simulink model "ds_fivezoneg36_backup"  (R2020a)
settings: Solver=ode1be  StartTime=182*24*3600  StopTime=183*24*3600  FixedStep=0.001  RelTol=1e-3
PostLoadFcn:
  | if any(exist('dsrtsu_mdlpostloadfcn', 'file') ~= 0), dsrtsu_mdlpostloadfcn('Execute', bdroot); end
InitFcn:
  | , if any(exist('rtifpga_mdlclblib', 'file') ~= 0), rtifpga_mdlclblib('Init', bdroot); end,
undefined symbols (not defined in the file or in its folder): dspaceexample_f_dy975f7hquM
libraries: neural x7
settings Model: DSRTSU_INTERNAL_RTI_VER=560  DSRTSU_INTERNAL_RTI_TYPE=rti1401  RTICANMMDATA=struct('GeneralSetupData',struct('modelroot','D:\github\dspace-modelica-example\dSpaceExample','generalsettings',struct('filesettings',struct('destfolder',struct('Name','RTICANMM_FILES','Check',1),'buildfolder',struct('Name','.','Check',1),'AbsDestfolder',struct('Name','D:\github\dspace-modelica-example\dSpaceExample\RTICANMM_FILES'),'AbsBuildfolder',struct('Name','D:\github\dspace-modelica-example\dSpaceExample'))),'options',struct('addpaths',1,'rmpaths',1,'addtrcexclusion',true,'cannavigator',struct('checkmonitoring',0),'show_usrtrc',0,'use_usrtrc',0),'advanced',struct('options',ones(1,100)),'MPSetup',{{}},'RTI',struct('Type','GRT','Ver','','Date',''),'modelname','ds_fivezoneg36','block','ds_fivezoneg36'))  DSRTSU_INTERNAL_RTIFPGA=160  Creator=yangyang.fu  LastModifiedBy=yangyang.fu
settings HardwareCC: TargetIntDivRoundTo=Zero  TargetEndianess=BigEndian  TargetHWDeviceType=Custom Processor->Custom
settings SFSimCC: MATLABDynamicMemAlloc=off
settings RTWCC: Description=Generic Real-Time Target  CustomInclude="\"C:\\Program Files\\Dymola 2021\\Source\""
settings GRTTargetCC: TargetLangStandard=C89/C90 (ANSI)

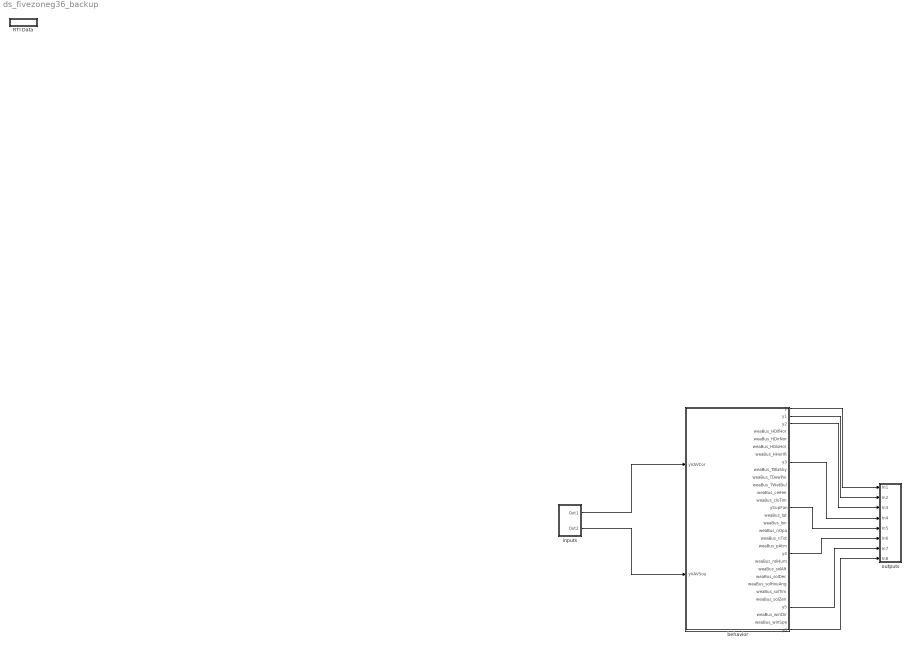
== system ds_fivezoneg36_backup ==
  RTI Data : Subsystem  Tag=struct('RTIDataServer',struct('RTIDataServerVs','2','RTIModelDescription','struct(''main'',''ds_fivezoneg36'',''sub'','''',''isMp'',0)'))  LoadFcn="if exist('rtidc'), try,  rtidc('DataHostBlockClbLoad', gcbh); catch, disp(['Warning: ''LoadFcn'' for RTI Data block failed: ' lasterr]); end, end,"  mask(RTI_DATA_HOST){}
      mask help:
      | RTI Data Block.
      | This block is used by RTI to store internal model-dependent data.
      | Please keep this block on the root level of the model. Deleting this block will result in data loss.
      |
      | NEVER DELETE OR COPY THIS BLOCK!
      settings: CopyFcn="if exist('rtidc'), try,  rtidc('DataHostBlockClbCopy', gcbh); catch, disp(['Warning: ''CopyFcn'' for RTI Data block failed: ' lasterr]); end, end,"  DeleteFcn="if exist('rtidc'), try,  rtidc('DataHostBlockClbDelete', gcbh); catch, disp(['Warning: ''DeleteFcn'' for RTI Data block failed: ' lasterr]); end, end,"  ModelCloseFcn="if exist('rtidc'), try,  rtidc('DataHostBlockClbModelClose', gcbh); catch, disp(['Warning: ''ModelCloseFcn'' for RTI Data block failed: ' lasterr]); end, end,"  PreSaveFcn="if exist('rtidc'), try,  rtidc('DataHostBlockClbPreSave', gcbh); catch, disp(['Warning: ''PreSaveFcn'' for RTI Data block failed: ' lasterr]); end, end,"  PostSaveFcn="if exist('rtidc'), try,  rtidc('DataHostBlockClbPostSave', gcbh); catch, disp(['Warning: ''PostSaveFcn'' for RTI Data block failed: ' lasterr]); end, end,"  NameChangeFcn="if exist('rtidc'), try,  rtidc('DataHostBlockClbNameChange', gcbh); catch, disp(['Warning: ''NameChangeFcn'' for RTI Data block failed: ' lasterr]); end, end,"
      mask Help:
      | RTI Data Block.
      | This block is used by RTI to store internal model-dependent data.
      | Please keep this block on the root level of the model. Deleting this block will result in data loss.
      | 
      | NEVER DELETE OR COPY THIS BLOCK!
      mask Display:
      | text(0.5, 0.5, 'RTI Data', 'HorizontalAlignment', 'center');
      | plot([1 0]);
  behavior : Subsystem
  inputs : Subsystem
  outputs : Subsystem
  wires:
  inputs/1(Out1) -> behavior/1(yVAVCor)
  inputs/2(Out2) -> behavior/2(yVAVSou)
  behavior/1(y) -> outputs/1(In1)
  behavior/2(y1) -> outputs/2(In2)
  behavior/3(y2) -> outputs/3(In3)
  behavior/8(y3) -> outputs/4(In4)
  behavior/14(ySupFan) -> outputs/5(In5)
  behavior/20(y4) -> outputs/6(In6)
  behavior/27(y5) -> outputs/7(In7)
  behavior/30(y6) -> outputs/8(In8)

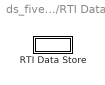
== system ds_fivezoneg36_backup/RTI Data ==
  RTI Data Store : Subsystem  Tag=struct('private',struct('version',struct('dsVer',uint32(2),'dsVerCreation',uint32(2),'RTI',struct('ver','7.14','type','RTI1401')),'access',struct('type','Model','isPerm',1,'created',['22-Sep-2021 20:42:39'],'modified',['29-Sep-2021 14:30:35'],'location','')),'public',struct('main',struct('data',[]),'sub',struct('name','','data',[])))  mask(RTI_DATA_STORE){}
      mask help:
      | RTI Data Store Block. This block is used by RTI to store internal model dependent data. Deleting this block will result in data loss.
      |
      | NEVER DELETE, COPY, OR MODIFY THIS BLOCK!
      mask Help:
      | RTI Data Store Block. This block is used by RTI to store internal model dependent data. Deleting this block will result in data loss.
      | 
      | NEVER DELETE, COPY, OR MODIFY THIS BLOCK!
      mask Display: text(0.5, 0.5, ' ', 'HorizontalAlignment', 'center');

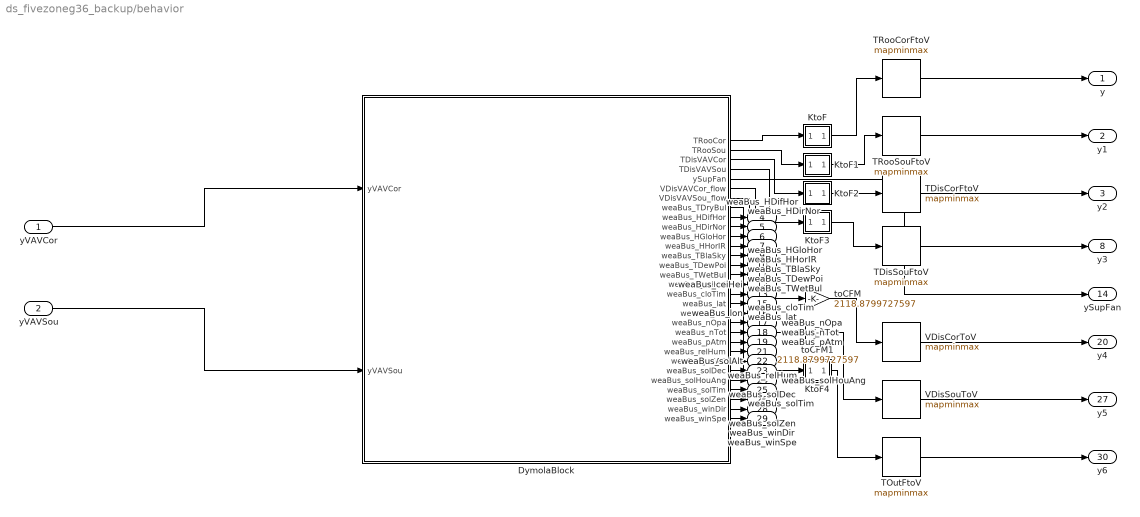
== system ds_fivezoneg36_backup/behavior ==
  yVAVCor : Inport
  yVAVSou : Inport  Port=2
  DymolaBlock : Subsystem  Tag=07-Sep-2021 15:30:30#975  LoadFcn=if exist('newDymolaGui') newDymolaGui('ds_fivezoneg36/behavior/DymolaBlock','PostLoadNew'); else error('Dymola not installed. Must install at least the file newDymolaGui.p'); end;
      mask help:
      | Dymola block.
      | A dymola block allows acausal physical modeling.
      | See Dymola manual for usage.
      settings: CopyFcn=newDymolaGui('07-Sep-2021 15:30:30#975','Copy');  DeleteFcn=if exist('newDymolaGui') newDymolaGui('ds_fivezoneg36/behavior/DymolaBlock','Delete'); end;  NameChangeFcn=newDymolaGui('07-Sep-2021 15:30:30#975','Copy');  OpenFcn=newDymolaGui('ds_fivezoneg36/behavior/DymolaBlock','Init');
      mask Display: image(reshape([1;1;1;1;1;1;1;1;1;1;1;1;1;1;1;1;1;1;1;1;1;1;0;0;0;0;0;0;0;0;0;0;1;1;1;1;1;1;1;1;0;1;1;1;1;1;1;1;1;0;1;1;1;1;1;0;0;0;0;0;0;0;1;1;0;0;0;0;0;0;0;1;1;0;0;0;0;0;0;0;1;1;0;0;0;0;0;0;0;1;1;0;0;0;0;0;0;0;1;1;0;0;0;0;0;0;0;1;1;0;0;0;0;0;0;0;1;1;0;0;0;0;0;0;0;1;1;0;0;0;0;0;0;0;1;1;0;0;0;0;0;0;0;1;1;0;0;0;0;0;0;0;1;1;0;0;0;0;0;0;0;1;1;0;0;0;0;0;0;0;1;1;0;0;0;0;0;0;0;1;1;0;0;0;0;0;0;0;1;1;0;0;0;0;0;0;0;1;1;0;0;0;0;0;0;0;1;1;0;0;0;0;0;0;0;1;1;0;0;0;0;0;0;0;1;1;0;0;0;0;0;0;0;1;1;0;0;0;0;0;0;0;1;1;0;0;0;0;0;0;0;1;1;0;0;0;0;0;0;0;1;1;0;0;0;0;0;0;0;1;1;1;1;1;0;1;1;1;1;1;1;1;1;0;1;1;1;1;1;1;1;1;0;0;0;0;0;0;0;0;0;0;1;1;1;1;1;1;1;1;1;1;1;1;1;1;1;1;1;1;1;1;1;1;1;1;1;1;1;1;1;1;1;1;1;1;1;1;1;1;1;1;1;1;1;1;0;0;0;0;0;0;0;0;0;0;1;1;1;1;1;1;1;1;0;1;1;1;1;1;1;1;1;0;1;1;1;1;1;0;0;0;0;0;0;0;1;1;0;0;0;0;0;0;0;1;1;0;0;0;0;0;0;0;1;1;0;0;0;0;0;0;0;1;1;0;0;0;0;0;0;0;1;1;0;0;0;0;0;0;0;1;1;0;0;0;0;0;0;0;1;1;0;0;0;0;0;0;0;1;1;0;0;0;0;0;0;0;1;1;0;0;0;0;0;0;0;1;1;0;0;0;0;0;0;0;1;1;0;0;0;0;0;0;0;1;1;0;0;0;0;0;0;0;1;1;0;0;0;0;0;0;0;1;1;0;0;0;0;0;0;0;1;1;0;0;0;0;0;0;0;1;1;0;0;0;0;0;0;0;1;1;0;0;0;0;0;0;0;1;1;0;0;0;0;0;0;0;1;1;0;0;0;0;0;0;0;1;1;0;0;0;0;0;0;0;1;1;0;0;0;0;0;0;0;1;1;0;0;0;0;0;0;0;1;1;0;0;0;0;0;0;0;1;1;1;1;1;0;1;1;1;1;1;1;1;1;0;1;1;1;1;1;1;1;1;0;0;0;0;0;0;0;0;0;0;1;1;1;1;1;1;1;1;1;1;1;1;1;1;1;1;1;1;1;1;1;1;1;1;1;1;1;1;1;1;1;1;1;1;1;1;1;1;1;1;1;1;1;1;0;0;0;0;0;0;0;0;0;0;1;1;1;1;1;1;1;1;0;1;1;1;1;1;1;1;1;0;1;1;1;1;1;0;0;0;0;0;0;0;1;1;0;0;0;0;0;0;0;1;1;0;1;1;1;1;1;0;1;1;0;1;1;1;1;1;0;1;1;0;1;1;1;1;1;0;1;1;0;1;1;1;1;1;0;1;1;0;1;1;1;1;1;0;1;1;0;1;1;1;1;1;0;1;1;0;1;1;1;1;1;0;1;1;0;1;1;1;1;1;0;1;1;0;1;1;1;1;1;0;1;1;0;1;1;1;1;1;0;1;1;0;1;1;1;1;1;0;1;1;0;1;1;1;1;1;0;1;1;0;1;1;1;1;1;0;1;1;0;1;1;1;1;1;0;1;1;0;1;1;1;1;1;0;1;1;0;1;1;1;1;1;0;1;1;0;1;1;1;1;1;0;1;1;0;1;1;1;1;1;0;1;1;0;1;1;1;1;1;0;1;1;0;1;1;1;1;1;0;1;1;0;0;0;0;0;0;0;1;1;0;0;0;0;0;0;0;1;1;1;1;1;0;1;1;1;1;1;1;1;1;0;1;1;1;1;1;1;1;1;0;0;0;0;0;0;0;0;0;0;1;1;1;1;1;1;1;1;1;1;1;1;1;1;1;1;1;1;1;1;1;1],18,18,3),[.2,.2,.6,.6])
  KtoF : Subsystem
  KtoF1 : Subsystem
  KtoF2 : Subsystem
  KtoF3 : Subsystem
  KtoF4 : Subsystem
  TDisCorFtoV : neural/Processing Functions/mapminmax  xmin=-150  xmax=150  ymin=-10  ymax=+10
  TDisSouFtoV : neural/Processing Functions/mapminmax  xmin=-150  xmax=150  ymin=-10  ymax=+10
  TOutFtoV : neural/Processing Functions/mapminmax  xmin=-150  xmax=150  ymin=-10  ymax=+10
  TRooCorFtoV : neural/Processing Functions/mapminmax  xmin=-150  xmax=150  ymin=-10  ymax=+10
  TRooSouFtoV : neural/Processing Functions/mapminmax  xmin=-150  xmax=150  ymin=-10  ymax=+10
  VDisCorToV : neural/Processing Functions/mapminmax  xmin=0  xmax=20000  ymin=-10  ymax=+10
  VDisSouToV : neural/Processing Functions/mapminmax  xmin=0  xmax=20000  ymin=-10  ymax=+10
  toCFM : Gain  Gain=2118.8799727597
  toCFM1 : Gain  Gain=2118.8799727597
  y : Outport
  y1 : Outport  Port=2
  y2 : Outport  Port=3
  weaBus_HDifHor : Outport  Port=4
  weaBus_HDirNor : Outport  Port=5
  weaBus_HGloHor : Outport  Port=6
  weaBus_HHorIR : Outport  Port=7
  y3 : Outport  Port=8
  weaBus_TBlaSky : Outport  Port=9
  weaBus_TDewPoi : Outport  Port=10
  weaBus_TWetBul : Outport  Port=11
  weaBus_ceiHei : Outport  Port=12
  weaBus_cloTim : Outport  Port=13
  ySupFan : Outport  Port=14
  weaBus_lat : Outport  Port=15
  weaBus_lon : Outport  Port=16
  weaBus_nOpa : Outport  Port=17
  weaBus_nTot : Outport  Port=18
  weaBus_pAtm : Outport  Port=19
  y4 : Outport  Port=20
  weaBus_relHum : Outport  Port=21
  weaBus_solAlt : Outport  Port=22
  weaBus_solDec : Outport  Port=23
  weaBus_solHouAng : Outport  Port=24
  weaBus_solTim : Outport  Port=25
  weaBus_solZen : Outport  Port=26
  y5 : Outport  Port=27
  weaBus_winDir : Outport  Port=28
  weaBus_winSpe : Outport  Port=29
  y6 : Outport  Port=30
  wires:
  DymolaBlock/17(weaBus_cloTim) -> weaBus_cloTim/1
  DymolaBlock/3(TDisVAVCor) -> KtoF2/1(In1)
  DymolaBlock/9(weaBus_HDifHor) -> weaBus_HDifHor/1
  DymolaBlock/28(weaBus_solZen) -> weaBus_solZen/1
  DymolaBlock/20(weaBus_nOpa) -> weaBus_nOpa/1
  DymolaBlock/7(VDisVAVSou_flow) -> toCFM1/1
  toCFM/1 -> VDisCorToV/1
  KtoF3/1(Out1) -> TDisSouFtoV/1
  DymolaBlock/8(weaBus_TDryBul) -> KtoF4/1(In1)
  DymolaBlock/4(TDisVAVSou) -> KtoF3/1(In1)
  DymolaBlock/19(weaBus_lon) -> weaBus_lon/1
  DymolaBlock/10(weaBus_HDirNor) -> weaBus_HDirNor/1
  TOutFtoV/1 -> y6/1
  DymolaBlock/6(VDisVAVCor_flow) -> toCFM/1
  DymolaBlock/13(weaBus_TBlaSky) -> weaBus_TBlaSky/1
  DymolaBlock/1(TRooCor) -> KtoF/1(In1)
  DymolaBlock/2(TRooSou) -> KtoF1/1(In1)
  TRooCorFtoV/1 -> y/1
  KtoF1/1(Out1) -> TRooSouFtoV/1
  KtoF4/1(Out1) -> TOutFtoV/1
  DymolaBlock/15(weaBus_TWetBul) -> weaBus_TWetBul/1
  KtoF2/1(Out1) -> TDisCorFtoV/1
  DymolaBlock/14(weaBus_TDewPoi) -> weaBus_TDewPoi/1
  toCFM1/1 -> VDisSouToV/1
  DymolaBlock/11(weaBus_HGloHor) -> weaBus_HGloHor/1
  KtoF/1(Out1) -> TRooCorFtoV/1
  DymolaBlock/5(ySupFan) -> ySupFan/1
  TRooSouFtoV/1 -> y1/1
  yVAVSou/1 -> DymolaBlock/2(yVAVSou)
  VDisSouToV/1 -> y5/1
  TDisCorFtoV/1 -> y2/1
  VDisCorToV/1 -> y4/1
  yVAVCor/1 -> DymolaBlock/1(yVAVCor)
  DymolaBlock/12(weaBus_HHorIR) -> weaBus_HHorIR/1
  DymolaBlock/18(weaBus_lat) -> weaBus_lat/1
  DymolaBlock/23(weaBus_relHum) -> weaBus_relHum/1
  DymolaBlock/29(weaBus_winDir) -> weaBus_winDir/1
  DymolaBlock/26(weaBus_solHouAng) -> weaBus_solHouAng/1
  DymolaBlock/16(weaBus_ceiHei) -> weaBus_ceiHei/1
  DymolaBlock/25(weaBus_solDec) -> weaBus_solDec/1
  DymolaBlock/21(weaBus_nTot) -> weaBus_nTot/1
  DymolaBlock/24(weaBus_solAlt) -> weaBus_solAlt/1
  DymolaBlock/30(weaBus_winSpe) -> weaBus_winSpe/1
  DymolaBlock/22(weaBus_pAtm) -> weaBus_pAtm/1
  DymolaBlock/27(weaBus_solTim) -> weaBus_solTim/1
  TDisSouFtoV/1 -> y3/1

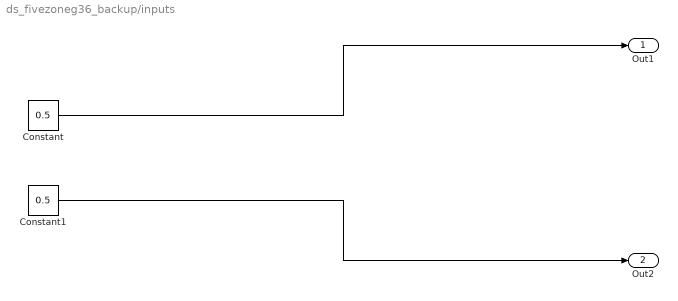
== system ds_fivezoneg36_backup/inputs ==
  Constant : Constant  Value=0.5  SampleTime=0.01
  Constant1 : Constant  Value=0.5  SampleTime=0.01
  Out1 : Outport
  Out2 : Outport  Port=2
  wires:
  Constant/1 -> Out1/1
  Constant1/1 -> Out2/1

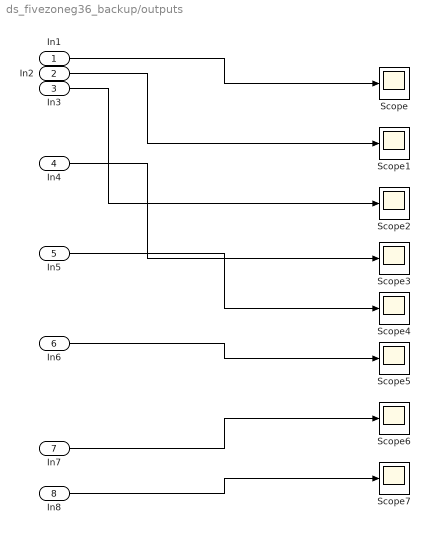
== system ds_fivezoneg36_backup/outputs ==
  In1 : Inport
  In2 : Inport  Port=2
  In3 : Inport  Port=3
  In4 : Inport  Port=4
  In5 : Inport  Port=5
  In6 : Inport  Port=6
  In7 : Inport  Port=7
  In8 : Inport  Port=8
  Scope{,1..7} (8 alike) : Scope
  wires:
  In4/1 -> Scope3/1
  In5/1 -> Scope4/1
  In2/1 -> Scope1/1
  In1/1 -> Scope/1
  In3/1 -> Scope2/1
  In8/1 -> Scope7/1
  In6/1 -> Scope5/1
  In7/1 -> Scope6/1

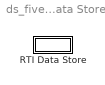
== system ds_fivezoneg36_backup/RTI Data/RTI Data Store ==
  RTI Data Store : Subsystem  mask(RTI_DATA_STORE){}
      mask help:
      | RTI Data Store Block. This block is used by RTI to store internal model dependent data. Deleting this block will result in data loss.
      |
      | NEVER DELETE, COPY, OR MODIFY THIS BLOCK!
      mask Help:
      | RTI Data Store Block. This block is used by RTI to store internal model dependent data. Deleting this block will result in data loss.
      | 
      | NEVER DELETE, COPY, OR MODIFY THIS BLOCK!
      mask Display: text(0.5, 0.5, ' ', 'HorizontalAlignment', 'center');

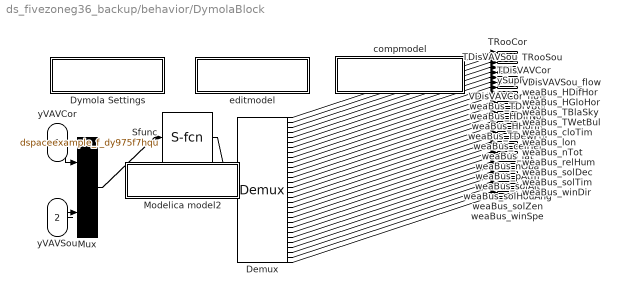
== system ds_fivezoneg36_backup/behavior/DymolaBlock ==
  yVAVCor : Inport
  yVAVSou : Inport  Port=2
  Demux : Demux  Outputs=[1;1;1;1;1;1;1;1;1;1;1;1;1;1;1;1;1;1;1;1;1;1;1;1;1;1;1;1;1;1]
  Dymola Settings : Subsystem  mask{ModelName=dSpaceExample.FiveZoneG36Demo, MoFileName=D:/github/dspace-modelica-example/dSpaceExample/FiveZoneG36Demo.mo, dSpace=, BusConnector=[], ResultFile=[], ResultFileOnline=[], ResultDt=[], Libs=:, bigobj=[], ImportFolder=[], guimode=[], ModelName2=[], forRuntime=[], MEXLoad=[], omitDescription=[], ResultName=ds_fivezoneg36}
      mask prompts: ModelName "Name of Dymola model"; MoFileName "File Name (including .mo)"; ResultFile "Create Result"; ResultFileOnline "Load result"; ResultDt "Result min dt"; Libs "Used Libraries"; bigobj "Compiler flag /bigobj"; ImportFolder "Import folder"; guimode "GUI mode flag"; ModelName2 "Model name for import mode"; forRuntime "Runtime export"; MEXLoad "Compiled S-function"; omitDescription "Omit description strings"; ResultName "Name of result file"
      mask Display: disp('Dymola Settings');
  Modelica model2 : Subsystem
      mask Display: disp('Change parameters');
  Mux : Mux  Inputs=[1;1]
  Sfunc : S-Function  Tag=975f7hqu  FunctionName=dspaceexample_f_dy975f7hqu  Parameters=[dspaceexample_f_dy975f7hquM.pV],[dspaceexample_f_dy975f7hquM.x0V]  PortCounts=[1;1]  SFunctionDeploymentMode=off  EnableBusSupport=off
      mask Display: image(imread('Dymola.bmp'))
  compmodel : Subsystem
      settings: OpenFcn=compileModelica('ds_fivezoneg36/behavior/DymolaBlock');
      mask Display: disp('Compile Modelica model');
  editmodel : Subsystem
      settings: OpenFcn=editModelica('ds_fivezoneg36/behavior/DymolaBlock');
      mask Display: disp('Edit Modelica model');
  TRooCor : Outport
  TRooSou : Outport  Port=2
  TDisVAVCor : Outport  Port=3
  TDisVAVSou : Outport  Port=4
  ySupFan : Outport  Port=5
  VDisVAVCor_flow : Outport  Port=6
  VDisVAVSou_flow : Outport  Port=7
  weaBus_TDryBul : Outport  Port=8
  weaBus_HDifHor : Outport  Port=9
  weaBus_HDirNor : Outport  Port=10
  weaBus_HGloHor : Outport  Port=11
  weaBus_HHorIR : Outport  Port=12
  weaBus_TBlaSky : Outport  Port=13
  weaBus_TDewPoi : Outport  Port=14
  weaBus_TWetBul : Outport  Port=15
  weaBus_ceiHei : Outport  Port=16
  weaBus_cloTim : Outport  Port=17
  weaBus_lat : Outport  Port=18
  weaBus_lon : Outport  Port=19
  weaBus_nOpa : Outport  Port=20
  weaBus_nTot : Outport  Port=21
  weaBus_pAtm : Outport  Port=22
  weaBus_relHum : Outport  Port=23
  weaBus_solAlt : Outport  Port=24
  weaBus_solDec : Outport  Port=25
  weaBus_solHouAng : Outport  Port=26
  weaBus_solTim : Outport  Port=27
  weaBus_solZen : Outport  Port=28
  weaBus_winDir : Outport  Port=29
  weaBus_winSpe : Outport  Port=30
  wires:
  Sfunc/1 -> Demux/1
  Demux/1 -> TRooCor/1
  Demux/2 -> TRooSou/1
  Demux/3 -> TDisVAVCor/1
  Demux/4 -> TDisVAVSou/1
  Demux/5 -> ySupFan/1
  Demux/6 -> VDisVAVCor_flow/1
  Demux/7 -> VDisVAVSou_flow/1
  Demux/8 -> weaBus_TDryBul/1
  Demux/9 -> weaBus_HDifHor/1
  Demux/10 -> weaBus_HDirNor/1
  Demux/11 -> weaBus_HGloHor/1
  Demux/12 -> weaBus_HHorIR/1
  Demux/13 -> weaBus_TBlaSky/1
  Demux/14 -> weaBus_TDewPoi/1
  Demux/15 -> weaBus_TWetBul/1
  Demux/16 -> weaBus_ceiHei/1
  Demux/17 -> weaBus_cloTim/1
  Demux/18 -> weaBus_lat/1
  Demux/19 -> weaBus_lon/1
  Demux/20 -> weaBus_nOpa/1
  Demux/21 -> weaBus_nTot/1
  Demux/22 -> weaBus_pAtm/1
  Demux/23 -> weaBus_relHum/1
  Demux/24 -> weaBus_solAlt/1
  Demux/25 -> weaBus_solDec/1
  Demux/26 -> weaBus_solHouAng/1
  Demux/27 -> weaBus_solTim/1
  Demux/28 -> weaBus_solZen/1
  Demux/29 -> weaBus_winDir/1
  Demux/30 -> weaBus_winSpe/1
  Mux/1 -> Sfunc/1
  yVAVCor/1 -> Mux/1
  yVAVSou/1 -> Mux/2

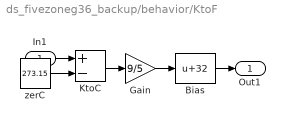
== system ds_fivezoneg36_backup/behavior/KtoF ==
  In1 : Inport
  Bias : Bias  Bias=32
  Gain : Gain  Gain=9/5
  KtoC : Sum  Inputs=+-
  zerC : Constant  Value=273.15  SampleTime=0
  Out1 : Outport
  wires:
  Gain/1 -> Bias/1
  KtoC/1 -> Gain/1
  zerC/1 -> KtoC/2
  Bias/1 -> Out1/1
  In1/1 -> KtoC/1

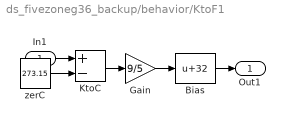
== system ds_fivezoneg36_backup/behavior/KtoF1 ==
  In1 : Inport
  Bias : Bias  Bias=32
  Gain : Gain  Gain=9/5
  KtoC : Sum  Inputs=+-
  zerC : Constant  Value=273.15  SampleTime=0
  Out1 : Outport
  wires:
  Gain/1 -> Bias/1
  KtoC/1 -> Gain/1
  zerC/1 -> KtoC/2
  Bias/1 -> Out1/1
  In1/1 -> KtoC/1

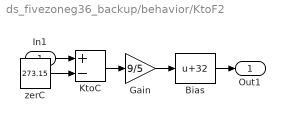
== system ds_fivezoneg36_backup/behavior/KtoF2 ==
  In1 : Inport
  Bias : Bias  Bias=32
  Gain : Gain  Gain=9/5
  KtoC : Sum  Inputs=+-
  zerC : Constant  Value=273.15  SampleTime=0
  Out1 : Outport
  wires:
  Gain/1 -> Bias/1
  KtoC/1 -> Gain/1
  zerC/1 -> KtoC/2
  Bias/1 -> Out1/1
  In1/1 -> KtoC/1

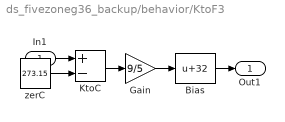
== system ds_fivezoneg36_backup/behavior/KtoF3 ==
  In1 : Inport
  Bias : Bias  Bias=32
  Gain : Gain  Gain=9/5
  KtoC : Sum  Inputs=+-
  zerC : Constant  Value=273.15  SampleTime=0
  Out1 : Outport
  wires:
  Gain/1 -> Bias/1
  KtoC/1 -> Gain/1
  zerC/1 -> KtoC/2
  Bias/1 -> Out1/1
  In1/1 -> KtoC/1

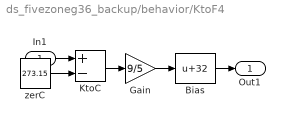
== system ds_fivezoneg36_backup/behavior/KtoF4 ==
  In1 : Inport
  Bias : Bias  Bias=32
  Gain : Gain  Gain=9/5
  KtoC : Sum  Inputs=+-
  zerC : Constant  Value=273.15  SampleTime=0
  Out1 : Outport
  wires:
  Gain/1 -> Bias/1
  KtoC/1 -> Gain/1
  zerC/1 -> KtoC/2
  Bias/1 -> Out1/1
  In1/1 -> KtoC/1

== system ds_fivezoneg36_backup/RTI Data/RTI Data Store/RTI Data Store ==
  RTI Data Store : Subsystem  mask(RTI_DATA_STORE){}
      mask help:
      | RTI Data Store Block. This block is used by RTI to store internal model dependent data. Deleting this block will result in data loss.
      |
      | NEVER DELETE, COPY, OR MODIFY THIS BLOCK!
      mask Help:
      | RTI Data Store Block. This block is used by RTI to store internal model dependent data. Deleting this block will result in data loss.
      | 
      | NEVER DELETE, COPY, OR MODIFY THIS BLOCK!
      mask Display: text(0.5, 0.5, ' ', 'HorizontalAlignment', 'center');

== system ds_fivezoneg36_backup/behavior/DymolaBlock/Dymola Settings ==

== system ds_fivezoneg36_backup/behavior/DymolaBlock/Modelica model2 ==

== system ds_fivezoneg36_backup/behavior/DymolaBlock/compmodel ==

== system ds_fivezoneg36_backup/behavior/DymolaBlock/editmodel ==

== system ds_fivezoneg36_backup/RTI Data/RTI Data Store/RTI Data Store/RTI Data Store ==
  RTI Data Store : Subsystem  mask(RTI_DATA_STORE){}
      mask help:
      | RTI Data Store Block. This block is used by RTI to store internal model dependent data. Deleting this block will result in data loss.
      |
      | NEVER DELETE, COPY, OR MODIFY THIS BLOCK!
      mask Help:
      | RTI Data Store Block. This block is used by RTI to store internal model dependent data. Deleting this block will result in data loss.
      | 
      | NEVER DELETE, COPY, OR MODIFY THIS BLOCK!
      mask Display: text(0.5, 0.5, ' ', 'HorizontalAlignment', 'center');

== system ds_fivezoneg36_backup/RTI Data/RTI Data Store/RTI Data Store/RTI Data Store/RTI Data Store ==
